simulink model "Simulation_Problem4"  (R2024a)
settings: Solver=ode15s  StartTime=0.0  StopTime=10.0  MaxStep=0.001  RelTol=1e-3
settings Model: Creator=hp  LastModifiedBy=hp

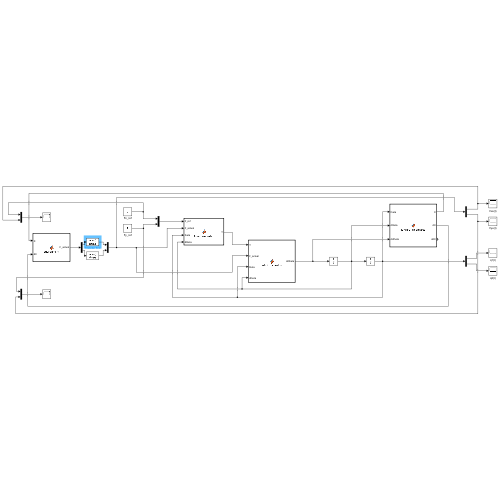
[thumbnail: Simulink's stored preview of the top-level diagram]
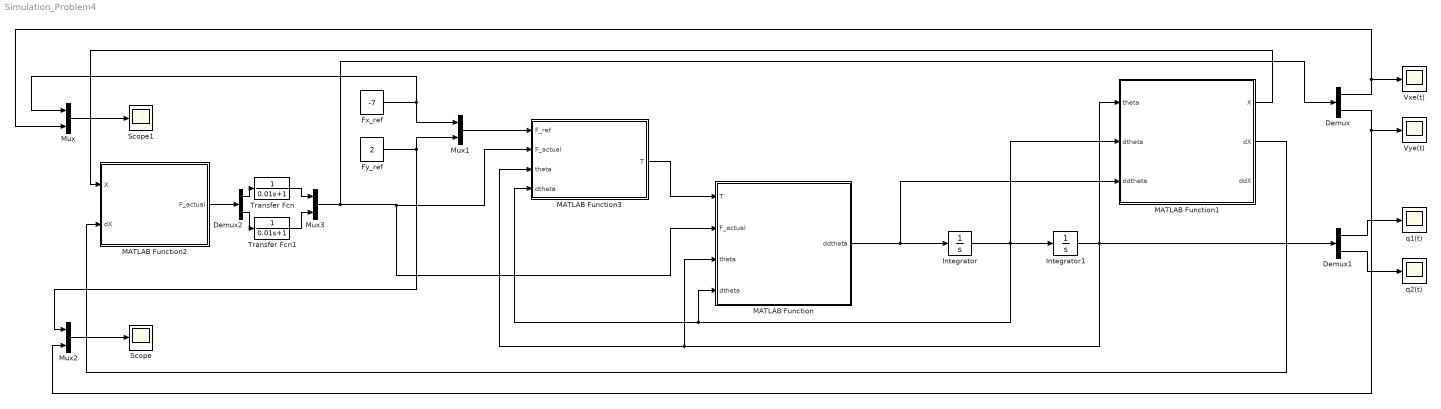
== system Simulation_Problem4 ==
  Demux : Demux  Outputs=2
  Demux1 : Demux  Outputs=2
  Demux2 : Demux  Outputs=2
  Fx_ref : Constant  Value=-7
  Fy_ref : Constant  Value=2
  Integrator : Integrator  InitialCondition=[0; 0]
  Integrator1 : Integrator  InitialCondition=[0; 0]
  MATLAB Function : MATLAB Function  TreatAsAtomicUnit=on
  MATLAB Function1 : MATLAB Function  TreatAsAtomicUnit=on
  MATLAB Function2 : MATLAB Function  TreatAsAtomicUnit=on
  MATLAB Function3 : MATLAB Function  TreatAsAtomicUnit=on
  Mux{,1..3} (4 alike) : Mux  Inputs=2
  Scope : Scope
  Scope1 : Scope
  Transfer Fcn : TransferFcn  Denominator=[0.01 1]
  Transfer Fcn1 : TransferFcn  Denominator=[0.01 1]
  Vxe(t) : Scope
  Vye(t) : Scope
  q1(t) : Scope
  q2(t) : Scope
  wires:
  Mux/1 -> Scope1/1
  MATLAB Function/1(ddtheta) -> Integrator/1, MATLAB Function1/3(ddtheta)
  Demux/1 -> Mux/2, Vxe(t)/1
  Mux2/1 -> Scope/1
  Demux1/1 -> q1(t)/1
  Demux1/2 -> q2(t)/1
  Demux/2 -> Mux2/2, Vye(t)/1
  MATLAB Function1/1(X) -> MATLAB Function2/1(X)
  MATLAB Function2/1(F_actual) -> Demux2/1
  Mux1/1 -> MATLAB Function3/1(F_ref)
  Fy_ref/1 -> Mux2/1, Mux1/2
  Fx_ref/1 -> Mux/1, Mux1/1
  MATLAB Function3/1(T) -> MATLAB Function/1(T)
  MATLAB Function1/2(dX) -> MATLAB Function2/2(dX)
  Mux3/1 -> Demux/1, MATLAB Function3/2(F_actual), MATLAB Function/2(F_actual)
  Integrator/1 -> MATLAB Function1/2(dtheta), MATLAB Function3/4(dtheta), MATLAB Function/4(dtheta), Integrator1/1
  Integrator1/1 -> MATLAB Function3/3(theta), MATLAB Function/3(theta), Demux1/1, MATLAB Function1/1(theta)
  Demux2/1 -> Transfer Fcn/1
  Demux2/2 -> Transfer Fcn1/1
  Transfer Fcn/1 -> Mux3/1
  Transfer Fcn1/1 -> Mux3/2

== matlab function Simulation_Problem4/MATLAB Function1 ==
  data: theta input; X output; dtheta input; ddtheta input; dX output; ddX output
function [X, dX, ddX] = forward_kinematics(theta, dtheta, ddtheta)
X = zeros(2,1); dX = zeros(2,1); ddX = zeros(2,1);
% Ileri Kinematik ve Jacobian Hesaplamalari

% l1 ve l2 degerleri
l1 = 0.83; 
l2 = 0.46;

th1 = theta(1); th2 = theta(2);
dth1 = dtheta(1); dth2 = dtheta(2);
ddth1 = ddtheta(1); ddth2 = ddtheta(2);

% 1. Konum (X)
xe = l1*cos(th1) + l2*cos(th1+th2);
ye = l1*sin(th1) + l2*sin(th1+th2);
X = [xe; ye];

% 2. Jacobian Matrisi ve Hiz (dX)
J11 = -l1*sin(th1) - l2*sin(th1+th2);
J12 = -l2*sin(th1+th2);
J21 = l1*cos(th1) + l2*cos(th1+th2);
J22 = l2*cos(th1+th2);
J = [J11, J12; J21, J22];

dX = J * [dth1; dth2];

% 3. Jacobian Turevi ve Ivme (ddX)
dJ11 = -l1*cos(th1)*dth1 - l2*cos(th1+th2)*(dth1+dth2);
dJ12 = -l2*cos(th1+th2)*(dth1+dth2);
dJ21 = -l1*sin(th1)*dth1 - l2*sin(th1+th2)*(dth1+dth2);
dJ22 = -l2*sin(th1+th2)*(dth1+dth2);
dJ = [dJ11, dJ12; dJ21, dJ22];

ddX = dJ * [dth1; dth2] + J * [ddth1; ddth2];
end

== matlab function Simulation_Problem4/MATLAB Function ==
  data: T input; F_actual input; ddtheta output; theta input; dtheta input
function ddtheta = robot_dynamics(T, F_actual, theta, dtheta)
ddtheta = zeros(2,1);
ddtheta = [0; 0];

% Kendi grubumuzun degerlerini garanti olsun diye buraya da yaziyoruz 
% (Simulink'in Workspace'den cekerken hata vermesini engellemek icin)
l1 = 0.83; l2 = 0.46;
r1 = 0.42; r2 = 0.23;
m1 = 0.66; m2 = 0.37;
I1 = 0.03; I2 = 0.02;
g = 9.81;

th1 = theta(1); th2 = theta(2);
dth1 = dtheta(1); dth2 = dtheta(2);
T1 = T(1); T2 = T(2);

% A(theta) Matrisi Parametreleri
a11 = m2*l1^2 + 2*m2*l1*r2*cos(th2) + m1*r1^2 + m2*r2^2 + I1 + I2; 
a12 = m2*r2^2 + l1*m2*r2*cos(th2) + I2; 
a21 = m2*r2^2 + l1*m2*r2*cos(th2) + I2; 
a22 = m2*r2^2 + I2; 
A = [a11, a12; a21, a22]; 

% B(theta, dtheta) Matrisi Parametreleri
b11 = -2*l1*m2*r2*sin(th2)*dth2; 
b12 = -2*l1*m2*r2*sin(th2)*dth1 - 2*l1*m2*r2*sin(th2)*dth2; 
b21 = 2*l1*m2*r2*sin(th2)*dth1; 
b22 = 0; 
B = [b11, b12; b21, b22]; 

% G(theta) Matrisi Parametreleri
g1 = m2*r2*g*cos(th1+th2) + m2*l1*g*cos(th1) + m1*r1*g*cos(th1); 
g2 = m2*r2*g*cos(th1+th2); 
G = [g1; g2]; 

% Jacobian Matrisi (Kuvveti eklemlere paylastirmak icin)
J11 = -l1*sin(th1) - l2*sin(th1+th2);
J12 = -l2*sin(th1+th2);
J21 = l1*cos(th1) + l2*cos(th1+th2);
J22 = l2*cos(th1+th2);
J = [J11, J12; J21, J22];

% Tork Vektoru
Tau = [T1; T2];

% Dinamik Denklemin Cozumu: ddtheta = A^-1 * (Tau - B*dtheta - G)
ddtheta = A \ (Tau - B*dtheta - G - J'*F_actual); 
end

== matlab function Simulation_Problem4/MATLAB Function2 ==
  data: X input; F_actual output; dX input
function F_actual = environment(X, dX)
% Problem 4 - Yay ve Damper Ortami

F_actual = [0; 0]; 

K_env = 650; % N/m
D_env = 120; % Ns/m
x_env = -0.1; 
y_env = 0.75; 

% X ekseninde duvara carpma sarti
if X(1) < x_env
    F_actual(1) = K_env * (X(1) - x_env) + D_env * dX(1);
end

% Y ekseninde duvara carpma sarti
if X(2) > y_env
    F_actual(2) = K_env * (X(2) - y_env) + D_env * dX(2);
end
end

== matlab function Simulation_Problem4/MATLAB Function3 ==
  data: F_ref input; T output; F_actual input; theta input; dtheta input
function T = force_controller(F_ref, F_actual, theta, dtheta)
T = [0; 0];

l1 = 0.83; l2 = 0.46;
m1 = 0.66; m2 = 0.37;
r1 = 0.42; r2 = 0.23;
g = 9.81;

th1 = theta(1); th2 = theta(2);

% Jacobian Matrisi
J11 = -l1*sin(th1) - l2*sin(th1+th2);
J12 = -l2*sin(th1+th2);
J21 = l1*cos(th1) + l2*cos(th1+th2);
J22 = l2*cos(th1+th2);
J = [J11, J12; J21, J22];

% G Matrisi (Yercekimi Kompanzasyonu)
g1 = m2*r2*g*cos(th1+th2) + m2*l1*g*cos(th1) + m1*r1*g*cos(th1);
g2 = m2*r2*g*cos(th1+th2);
G = [g1; g2];

% Kontrol Katsayilari 
Kf = 1.5; 
Kd = 10; 

% Uygulanacak Hedef Tork: T = J^T * (F_ref + P_Kontrol) + G - Hiz_Sonumleme
F_cmd = F_ref + Kf * (F_ref - F_actual);
T = J' * F_cmd + G - Kd * dtheta;
end
